simulink model "Lab2_Transient"  (R2016a)
settings: Solver=VariableStepAuto  StartTime=0.0  StopTime=30  RelTol=1e-3
settings Model: Creator=jordan  LastModifiedBy=jordan

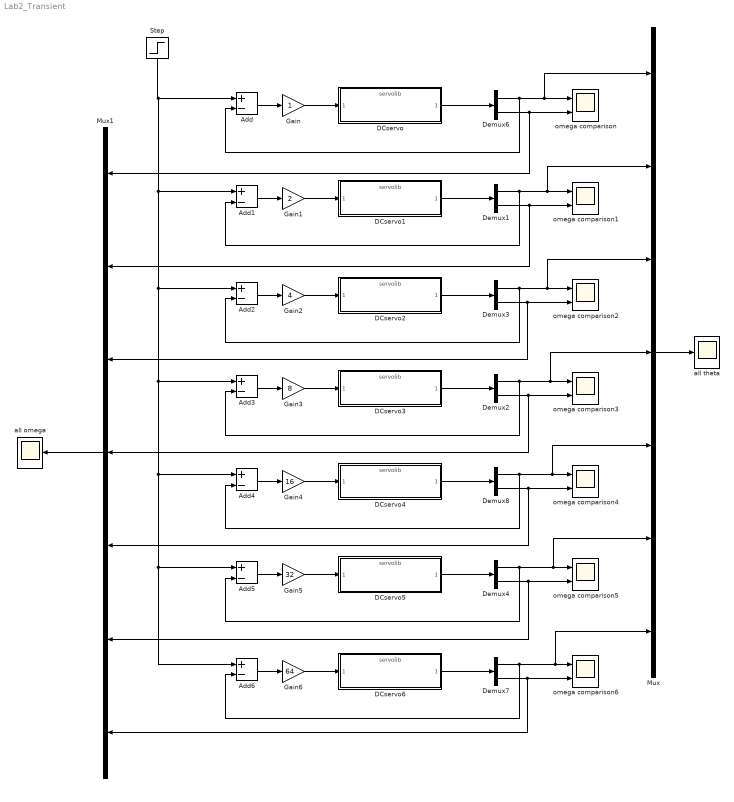
== system Lab2_Transient ==
  Add{,1..6} (7 alike) : Sum  Inputs=+-
  DCservo{,1..6} (7 alike) : ModelReference  ModelNameDialog=servolib.slx  SimulationMode=Normal  ModelReferenceVersion=1.71
  Demux{1..4,6..8} (7 alike) : Demux  Outputs=2
  Gain : Gain
  Gain1 : Gain  Gain=2
  Gain2 : Gain  Gain=4
  Gain3 : Gain  Gain=8
  Gain4 : Gain  Gain=16
  Gain5 : Gain  Gain=32
  Gain6 : Gain  Gain=64
  Mux : Mux  Inputs=7
  Mux1 : Mux  Inputs=7
  Step : Step  SampleTime=0
  all omega : Scope
  all theta : Scope
  omega comparison{,1..6} (7 alike) : Scope  NumInputPorts=2
  wires:
  Demux6/2 -> Mux1/1, omega comparison/2
  Demux6/1 -> Add/2, Mux/1, omega comparison/1
  DCservo/1 -> Demux6/1
  Step/1 -> Add/1, Add1/1, Add2/1, Add3/1, Add4/1, Add5/1, Add6/1
  Add/1 -> Gain/1
  Gain/1 -> DCservo/1
  Demux1/2 -> Mux1/2, omega comparison1/2
  DCservo1/1 -> Demux1/1
  Add1/1 -> Gain1/1
  Gain1/1 -> DCservo1/1
  Demux3/2 -> Mux1/3, omega comparison2/2
  Demux3/1 -> Add2/2, Mux/3, omega comparison2/1
  DCservo2/1 -> Demux3/1
  Add2/1 -> Gain2/1
  Gain2/1 -> DCservo2/1
  Demux2/2 -> Mux1/4, omega comparison3/2
  Demux2/1 -> Add3/2, Mux/4, omega comparison3/1
  DCservo3/1 -> Demux2/1
  Add3/1 -> Gain3/1
  Gain3/1 -> DCservo3/1
  Demux8/2 -> Mux1/5, omega comparison4/2
  Demux8/1 -> Add4/2, Mux/5, omega comparison4/1
  DCservo4/1 -> Demux8/1
  Add4/1 -> Gain4/1
  Gain4/1 -> DCservo4/1
  Demux4/2 -> Mux1/6, omega comparison5/2
  Demux4/1 -> Add5/2, Mux/6, omega comparison5/1
  DCservo5/1 -> Demux4/1
  Add5/1 -> Gain5/1
  Gain5/1 -> DCservo5/1
  Demux7/2 -> Mux1/7, omega comparison6/2
  Demux7/1 -> Add6/2, Mux/7, omega comparison6/1
  DCservo6/1 -> Demux7/1
  Add6/1 -> Gain6/1
  Gain6/1 -> DCservo6/1
  Demux1/1 -> Add1/2, Mux/2, omega comparison1/1
  Mux/1 -> all theta/1
  Mux1/1 -> all omega/1
